simulink model "PCS_Grid_Connection_v3"  (R2025a)
settings: Solver=ode4  StartTime=0.0  StopTime=0.5  FixedStep=1e-5  RelTol=1e-3
Description:
  | PCS Grid-Connected Simulation Results
  | Parameters: Vgrid=220Vrms, L=5.0mH, R=0.1 Ohm, f=50Hz
  | Equation: L*di/dt = Vpcs - Vgrid - R*i
  | ---------------------------------------------------------------
  | Case                         P(W)       Q(var)     I_rms(A) State
  | ---------------------------------------------------------------
  | 0 deg (同幅)                    0.0          0.0         0.00 -, -
  | 10 deg                     5299.1        805.4        24.36 输出有功, 输出无功(容性)
  | 45 deg                    21126.7      10369.7       106.97 输出有功, 输出无功(容性)
  | 90 deg                    28731.8      32641.5       197.66 输出有功, 输出无功(容性)
  | 135 deg                   18360.3      53769.0       258.26 输出有功, 输出无功(容性)
  | 180 deg                   -3912.3      61375.8       279.55 吸收有功, 输出无功(容性)
  | -45 deg                  -22272.5       7607.0       106.98 吸收有功, 输出无功(容性)
  | -90 deg                  -32643.9      28734.5       197.68 吸收有功, 输出无功(容性)
  | Vp=230V,0 deg (感性示例)         88.9      -1394.9         6.35 输出有功, 吸收无功(感性)
  | ---------------------------------------------------------------
  | Key findings:
  | 1. Vpcs=Vgrid with phase sweep: current mostly capacitive (Q>0) due to
  |    inductor impedance angle (86.4 deg) rotating the voltage difference vector.
  | 2. Inductive state (Q<0) requires Vpcs amplitude slightly above Vgrid (~230V)
  |    with near-zero phase difference.
  | 3. P sign determined by PCS phase vs Grid. Q sign depends on both amplitude and phase.
settings Model: Creator=jicai  LastModifiedBy=jicai

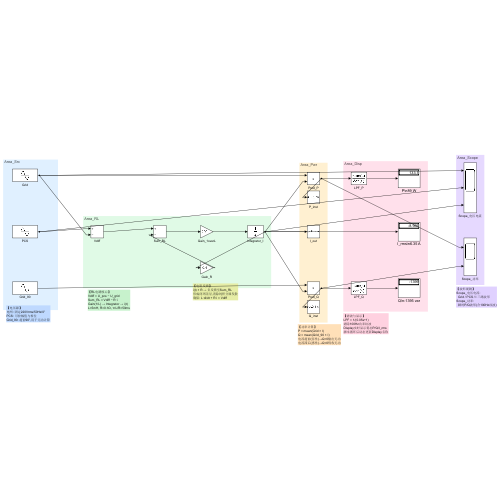
[thumbnail: Simulink's stored preview of the top-level diagram]
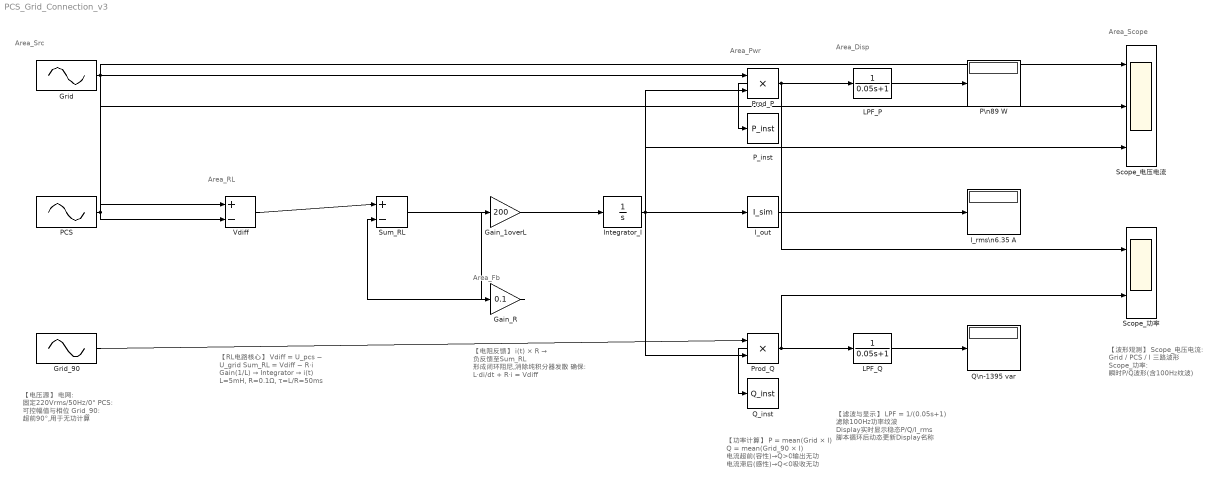
== system PCS_Grid_Connection_v3 ==
  note: Area_Src
  note: Area_RL
  note: Area_Pwr
  note: Area_Disp
  note: Area_Scope
  note: Area_Fb
  note: 【电压源】
      | 电网: 固定220Vrms/50Hz/0°
      | PCS: 可控幅值与相位
      | Grid_90: 超前90°,用于无功计算
  note: 【RL电路核心】
      | Vdiff = U_pcs − U_grid
      | Sum_RL = Vdiff − R·i
      | Gain(1/L) → Integrator → i(t)
      | L=5mH, R=0.1Ω, τ=L/R=50ms
  note: 【功率计算】
      | P = mean(Grid × I)
      | Q = mean(Grid_90 × I)
      | 电流超前(容性)→Q>0输出无功
      | 电流滞后(感性)→Q<0吸收无功
  note: 【滤波与显示】
      | LPF = 1/(0.05s+1)
      | 滤除100Hz功率纹波
      | Display实时显示稳态P/Q/I_rms
      | 脚本循环后动态更新Display名称
  note: 【波形观测】
      | Scope_电压电流:
      |   Grid / PCS / I 三路波形
      | Scope_功率:
      |   瞬时P/Q波形(含100Hz纹波)
  note: 【电阻反馈】
      | i(t) × R → 负反馈至Sum_RL
      | 形成闭环阻尼,消除纯积分器发散
      | 确保: L·di/dt + R·i = Vdiff
  Gain_1overL : Gain  Gain=200
  Gain_R : Gain  Gain=0.1
  Grid : Sin  Amplitude=311.127  Frequency=314.1593  SampleTime=0
  Grid_90 : Sin  Amplitude=311.127  Frequency=314.1593  Phase=1.5708  SampleTime=0
  I_out : ToWorkspace  VariableName=I_sim  SampleTime=-1
  I_rms\n6.35 A : Display
  Integrator_I : Integrator
  LPF_P : TransferFcn  Denominator=[0.05 1]
  LPF_Q : TransferFcn  Denominator=[0.05 1]
  PCS : Sin  Amplitude=325.2691  Frequency=314.1593  SampleTime=0
  P\n89 W : Display
  P_inst : ToWorkspace  VariableName=P_inst  SampleTime=-1
  Prod_P : Product
  Prod_Q : Product
  Q\n-1395 var : Display
  Q_inst : ToWorkspace  VariableName=Q_inst  SampleTime=-1
  Scope_功率 : Scope  NumInputPorts=2
  Scope_电压电流 : Scope  NumInputPorts=3
  Sum_RL : Sum  Inputs=+-
  Vdiff : Sum  Inputs=+-
  wires:
  PCS/1 -> Vdiff/1, Scope_电压电流/2
  Grid/1 -> Vdiff/2, Prod_P/1, Scope_电压电流/1
  Vdiff/1 -> Sum_RL/1
  Sum_RL/1 -> Gain_1overL/1
  Gain_1overL/1 -> Integrator_I/1
  Integrator_I/1 -> Gain_R/1, Prod_P/2, I_out/1, I_rms\n6.35 A/1, Prod_Q/2, Scope_电压电流/3
  Gain_R/1 -> Sum_RL/2
  Prod_P/1 -> P_inst/1, LPF_P/1, Scope_功率/1
  LPF_P/1 -> P\n89 W/1
  Grid_90/1 -> Prod_Q/1
  Prod_Q/1 -> Q_inst/1, LPF_Q/1, Scope_功率/2
  LPF_Q/1 -> Q\n-1395 var/1
